simulink model "Plant"  (R2015a)
settings: Solver=ode3  StartTime=0.0  StopTime=10.0  FixedStep=0.001  RelTol=1e-3
settings Model: Creator=GeoLee  LastModifiedBy=geolee

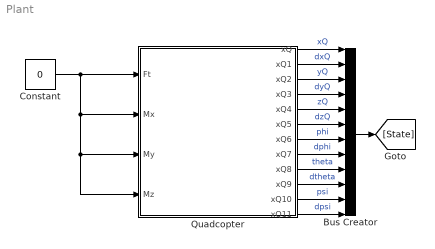
== system Plant ==
  Bus Creator : BusCreator  Inputs=12
  Constant : Constant  Value=0
  Quadcopter : Subsystem  mask(Single Quadcopter Plant){x0=0, y0=0, z0=0}
      mask prompts: x0 "Initial position of x (m)"; y0 "Initial position of y (m)"; z0 "Initial position of z (m)"
      mask help:
      | Attention:
      | the first input Ft is actually dF!
      mask Display:
      | image('Quad_pic.png');
      | port_label('input', 1, 'Ft');
      | port_label('input', 2, 'Mx');
      | port_label('input', 3, 'My');
      | port_label('input', 4, 'Mz');
      | port_label('output', 1, 'xQ');
      | port_label('output', 2, 'dxQ');
      | port_label('output', 3, 'yQ');
      | port_label('output', 4, 'dyQ');
      | port_label('output', 5, 'zQ');
      | port_label('output', 6, 'dzQ');
      | port_label('output', 7, 'phi');
      | port_label('output', 8, 'dphi');
      | port_label('output', 9, 'theta');
      | port_label('output', 10, 'dtheta');
      | port_label('output', 11, 'psi');
      | port_label('output', 12, 'dpsi');
  wires:
  Quadcopter/6(xQ5) -> Bus Creator/6  "dzQ"
  Quadcopter/5(xQ4) -> Bus Creator/5  "zQ"
  Quadcopter/7(xQ6) -> Bus Creator/7  "phi"
  Quadcopter/4(xQ3) -> Bus Creator/4  "dyQ"
  Quadcopter/8(xQ7) -> Bus Creator/8  "dphi"
  Quadcopter/3(xQ2) -> Bus Creator/3  "yQ"
  Quadcopter/9(xQ8) -> Bus Creator/9  "theta"
  Quadcopter/2(xQ1) -> Bus Creator/2  "dxQ"
  Quadcopter/10(xQ9) -> Bus Creator/10  "dtheta"
  Quadcopter/11(xQ10) -> Bus Creator/11  "psi"
  Quadcopter/1(xQ) -> Bus Creator/1  "xQ"
  Quadcopter/12(xQ11) -> Bus Creator/12  "dpsi"
  Bus Creator/1 -> [State]
  Constant/1 -> Quadcopter/2(Mx), Quadcopter/3(My), Quadcopter/4(Mz), Quadcopter/1(Ft)

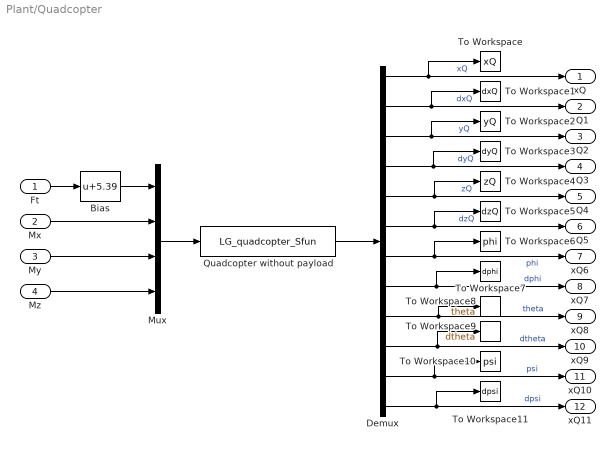
== system Plant/Quadcopter ==
  Ft : Inport
  Mx : Inport  Port=2
  My : Inport  Port=3
  Mz : Inport  Port=4
  Bias : Bias  Bias=5.39
  Demux : Demux  Outputs=12
  Mux : Mux
  Quadcopter without payload : S-Function  FunctionName=LG_quadcopter_Sfun  Parameters=x0,y0,z0
  To Workspace : ToWorkspace  VariableName=xQ  SampleTime=-1
  To Workspace1 : ToWorkspace  VariableName=dxQ  SampleTime=-1
  To Workspace10 : ToWorkspace  VariableName=psi  SampleTime=-1
  To Workspace11 : ToWorkspace  VariableName=dpsi  SampleTime=-1
  To Workspace2 : ToWorkspace  VariableName=yQ  SampleTime=-1
  To Workspace3 : ToWorkspace  VariableName=dyQ  SampleTime=-1
  To Workspace4 : ToWorkspace  VariableName=zQ  SampleTime=-1
  To Workspace5 : ToWorkspace  VariableName=dzQ  SampleTime=-1
  To Workspace6 : ToWorkspace  VariableName=phi  SampleTime=-1
  To Workspace7 : ToWorkspace  VariableName=dphi  SampleTime=-1
  To Workspace8 : ToWorkspace  VariableName=theta  SampleTime=-1
  To Workspace9 : ToWorkspace  VariableName=dtheta  SampleTime=-1
  xQ : Outport
  xQ1 : Outport  Port=2
  xQ2 : Outport  Port=3
  xQ3 : Outport  Port=4
  xQ4 : Outport  Port=5
  xQ5 : Outport  Port=6
  xQ6 : Outport  Port=7
  xQ7 : Outport  Port=8
  xQ8 : Outport  Port=9
  xQ9 : Outport  Port=10
  xQ10 : Outport  Port=11
  xQ11 : Outport  Port=12
  wires:
  Mux/1 -> Quadcopter without payload/1
  Ft/1 -> Bias/1
  Quadcopter without payload/1 -> Demux/1
  Mz/1 -> Mux/4
  Bias/1 -> Mux/1
  Demux/9 -> To Workspace8/1, xQ8/1  "theta"
  Demux/1 -> xQ/1, To Workspace/1  "xQ"
  Demux/7 -> xQ6/1, To Workspace6/1  "phi"
  Demux/11 -> xQ10/1, To Workspace10/1  "psi"
  Demux/4 -> xQ3/1, To Workspace3/1  "dyQ"
  Demux/2 -> xQ1/1, To Workspace1/1  "dxQ"
  Demux/3 -> xQ2/1, To Workspace2/1  "yQ"
  Demux/10 -> xQ9/1, To Workspace9/1  "dtheta"
  Demux/5 -> xQ4/1, To Workspace4/1  "zQ"
  Demux/8 -> xQ7/1, To Workspace7/1  "dphi"
  Demux/12 -> xQ11/1, To Workspace11/1  "dpsi"
  Demux/6 -> xQ5/1, To Workspace5/1  "dzQ"
  My/1 -> Mux/3
  Mx/1 -> Mux/2
